simulink model "PFE_2Lignes_RNA (2)"  (R2024a)
settings: Solver=ode4  StartTime=0.0  StopTime=0.18  RelTol=1e-3
libraries: neural x202, spsRMSLib x12, spsThreePhasePISectionLineLib x4, spsThreePhaseFaultLib x2, spsThreePhaseVIMeasurementLib x2, spsThreePhaseSourceLib x2, spspowerguiLib x1
(part 5 of 10)

== system PFE_2Lignes_RNA (2)/RNA_Classificateur/Layer 3/Delays 1 ==
  "p{3}" : Inport  PortDimensions=20
      mask Display: e = 0.06;c1 = [120 230 180]/255;c2 = ([120 230 180]+0)/(256+128);c3 = ([120 230 180]+128)/(256+128);patch([0 1 1 0],[0 0 1 1],c1);patch([0 1 1 1-e 1-e 0+e],[0 0 1 1-e 0+e 0+e],c2);patch([0 0 1 1-e 0+e 0+e],[0 1 1 1-e 1-e 0+e],c3);plot([0 1 1 0 0],[0 0 1 1 0]);
  mux : Mux  Inputs=1
      mask Display: e = 0.06;c1 = [120 150 230]/255;c2 = ([120 150 230]+0)/383;c3 = ([120 150 230]+128)/383;patch([0 1 1 0],[0 0 1 1],c1);patch([0 1 1 1-e 1-e 0+e],[0 0 1 1-e 0+e 0+e],c2);patch([0 0 1 1-e 0+e 0+e],[0 1 1 1-e 1-e 0+e],c3);plot([0 1 1 0 0],[0 0 1 1 0]);disp('Mux')
  "pd{3,2}" : Outport
      mask Display: e = 0.06;c1 = [120 230 180]/255;c2 = ([120 230 180]+0)/(256+128);c3 = ([120 230 180]+128)/(256+128);patch([0 1 1 0],[0 0 1 1],c1);patch([0 1 1 1-e 1-e 0+e],[0 0 1 1-e 0+e 0+e],c2);patch([0 0 1 1-e 0+e 0+e],[0 1 1 1-e 1-e 0+e],c3);plot([0 1 1 0 0],[0 0 1 1 0]);
  wires:
  "p{3}"/1 -> mux/1
  mux/1 -> "pd{3,2}"/1

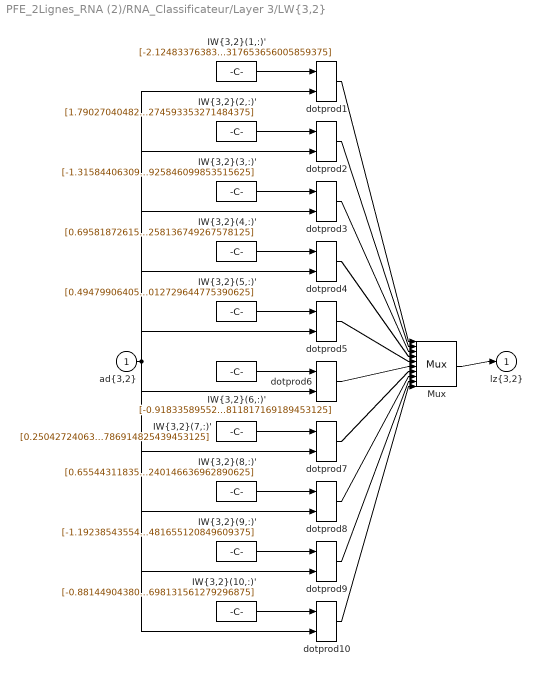
== system PFE_2Lignes_RNA (2)/RNA_Classificateur/Layer 3/LW{3,2} ==
  "ad{3,2}" : Inport  PortDimensions=20
      mask Display: e = 0.06;c1 = [120 230 180]/255;c2 = ([120 230 180]+0)/(256+128);c3 = ([120 230 180]+128)/(256+128);patch([0 1 1 0],[0 0 1 1],c1);patch([0 1 1 1-e 1-e 0+e],[0 0 1 1-e 0+e 0+e],c2);patch([0 0 1 1-e 0+e 0+e],[0 1 1 1-e 1-e 0+e],c3);plot([0 1 1 0 0],[0 0 1 1 0]);
  "IW{3,2}(1,:)'" : Constant  Value=[-2.124833763838835043458175277919508516788482666015625;2.235095062674105736988394710351713001728057861328125;-1.495799673223132675303759242524392902851104736328125;-0.10326184150683544171744898676479351706802845001220703125;0.30461440661710204036438653929508291184902191162109375;1.7655833119941684028475492596044205129146575927734375;-0.294301775431359435852840533698326908051967620849609375;1.422921443728915935622580946073867380619049072265625;-1.0126081617278674951165839956956915557384490966796875;2.06139005636338179527911051991395652294158935546875;-1.42107797840496008490163148962892591953277587890625;-0.4665987521331393939050258268252946436405181884765625;-0.78123086378600870016697399478289298713207244873046875;-0.9638905255282874673383730623754672706127166748046875;0.11887587911221302039432856645362335257232189178466796875;0.1219190321385441311274888676052796654403209686279296875;0.7209704057204142646497757596080191433429718017578125;0.807266197382073169563909686985425651073455810546875;-1.1797771643987851053481108465348370373249053955078125;-0.2368631238857614729198530767462216317653656005859375]
      mask Display: e = 0.06;c1 = [120 150 230]/255;c2 = ([120 150 230]+0)/383;c3 = ([120 150 230]+128)/383;patch([0 1 1 0],[0 0 1 1],c1);patch([0 1 1 1-e 1-e 0+e],[0 0 1 1-e 0+e 0+e],c2);patch([0 0 1 1-e 0+e 0+e],[0 1 1 1-e 1-e 0+e],c3);plot([0 1 1 0 0],[0 0 1 1 0]);disp('weights');
  "IW{3,2}(10,:)'" : Constant  Value=[-0.88144904380601041271603435234283097088336944580078125;1.2959793842845128697405243656248785555362701416015625;1.3513640222311844585334483781480230391025543212890625;-0.44568678579454512611590644155512563884258270263671875;-0.485414780167485904183166667280602268874645233154296875;-0.7871810260425171623666074083303101360797882080078125;2.007996352418774943515700215357355773448944091796875;-0.37565487427648835971893959140288643538951873779296875;-1.0046399001899637415391453032498247921466827392578125;-0.64463016403909667584315457133925519883632659912109375;1.4514250561273047690491466710227541625499725341796875;-1.64089130459730281330621437518857419490814208984375;0.85543383350244595053624152569682337343692779541015625;0.266300186174826258866943362590973265469074249267578125;1.525362775288933381290235047345049679279327392578125;-1.0373978509685557458652738205273635685443878173828125;-0.189926019352055830413661396960378624498844146728515625;-0.51200224756051238017562354798428714275360107421875;0.72520479466617115971160956178209744393825531005859375;1.131488984637971650926147049176506698131561279296875]
      mask Display: e = 0.06;c1 = [120 150 230]/255;c2 = ([120 150 230]+0)/383;c3 = ([120 150 230]+128)/383;patch([0 1 1 0],[0 0 1 1],c1);patch([0 1 1 1-e 1-e 0+e],[0 0 1 1-e 0+e 0+e],c2);patch([0 0 1 1-e 0+e 0+e],[0 1 1 1-e 1-e 0+e],c3);plot([0 1 1 0 0],[0 0 1 1 0]);disp('weights');
  "IW{3,2}(2,:)'" : Constant  Value=[1.7902704048235531519850383119774051010608673095703125;-0.83301117298299443003628539372584782540798187255859375;-0.86812317640997616052800367469899356365203857421875;-0.61903270694970424781189421992166899144649505615234375;-1.0952786106124217102575357785099186003208160400390625;0.98637534583504626883865284980856813490390777587890625;2.1858479023867385393486983957700431346893310546875;0.967325919819800095211803636630065739154815673828125;0.75786317317939388971126390970312058925628662109375;-2.060200915980545222083719636430032551288604736328125;-1.4236157537296836306239811165141873061656951904296875;1.2433599401893744573754929660935886204242706298828125;0.05806739015085897459567121359214070253074169158935546875;0.0020380782368509021973412842498873942531645298004150390625;0.84058335857627441978223714613704942166805267333984375;1.35282448767321827887144536362029612064361572265625;0.2189926893955626285848126144628622569143772125244140625;-0.42231741579335657643667900629225187003612518310546875;1.436115452384581825384657349786721169948577880859375;-0.41474159462432014233712607165216468274593353271484375]
      mask Display: e = 0.06;c1 = [120 150 230]/255;c2 = ([120 150 230]+0)/383;c3 = ([120 150 230]+128)/383;patch([0 1 1 0],[0 0 1 1],c1);patch([0 1 1 1-e 1-e 0+e],[0 0 1 1-e 0+e 0+e],c2);patch([0 0 1 1-e 0+e 0+e],[0 1 1 1-e 1-e 0+e],c3);plot([0 1 1 0 0],[0 0 1 1 0]);disp('weights');
  "IW{3,2}(3,:)'" : Constant  Value=[-1.3158440630983820884836177356191910803318023681640625;-1.419656511869585191476517138653434813022613525390625;1.1800655789785725602314414572902023792266845703125;-0.719240970988912042827223558560945093631744384765625;-0.11943453151677159429500107989952084608376026153564453125;-1.9966258446750460020524542414932511746883392333984375;-2.37447351454145749727331349276937544345855712890625;-0.78258770171416525140983821984264068305492401123046875;1.0354694090954545959704091728781349956989288330078125;0.605154989361207373832485245657153427600860595703125;1.23491208175254296719458579900674521923065185546875;1.2582457853531112679235093310126103460788726806640625;-0.67352823452173193885528235114179551601409912109375;0.85550010884744087658049238598323427140712738037109375;-1.2449073010859830201724207654478959739208221435546875;-0.449245519413075999892726031248457729816436767578125;0.07641744133077221778904686289024539291858673095703125;-0.426118641723025659562296141302795149385929107666015625;1.7786706927411055634280501180910505354404449462890625;-0.68789532767131744694921735572279430925846099853515625]
      mask Display: e = 0.06;c1 = [120 150 230]/255;c2 = ([120 150 230]+0)/383;c3 = ([120 150 230]+128)/383;patch([0 1 1 0],[0 0 1 1],c1);patch([0 1 1 1-e 1-e 0+e],[0 0 1 1-e 0+e 0+e],c2);patch([0 0 1 1-e 0+e 0+e],[0 1 1 1-e 1-e 0+e],c3);plot([0 1 1 0 0],[0 0 1 1 0]);disp('weights');
  "IW{3,2}(4,:)'" : Constant  Value=[0.69581872615161532991123749525286257266998291015625;-2.475637159212695781462798549910075962543487548828125;-1.0133208738240877533343109462293796241283416748046875;0.433411808461749981091770678176544606685638427734375;1.437967549207739725858345991582609713077545166015625;2.081675820617252536948171837138943374156951904296875;0.52801372365134557895771649782545864582061767578125;1.610670852459428648018047169898636639118194580078125;0.424212418998134166425728608373901806771755218505859375;1.6976510238713957701151002765982411801815032958984375;-0.08330331033522976602601062268149689771234989166259765625;-0.2255126598263615667061543490490294061601161956787109375;-0.5215191203851128332047437652363441884517669677734375;0.8126804349301448571196715420228429138660430908203125;-1.1216344746556570211026837569079361855983734130859375;0.80258429428750144296600410598330199718475341796875;-0.149635019068319385926457698587910272181034088134765625;0.7331158653688760740152474681963212788105010986328125;-2.20447234463556807071427101618610322475433349609375;0.10647105238430194795729022416708176024258136749267578125]
      mask Display: e = 0.06;c1 = [120 150 230]/255;c2 = ([120 150 230]+0)/383;c3 = ([120 150 230]+128)/383;patch([0 1 1 0],[0 0 1 1],c1);patch([0 1 1 1-e 1-e 0+e],[0 0 1 1-e 0+e 0+e],c2);patch([0 0 1 1-e 0+e 0+e],[0 1 1 1-e 1-e 0+e],c3);plot([0 1 1 0 0],[0 0 1 1 0]);disp('weights');
  "IW{3,2}(5,:)'" : Constant  Value=[0.4947990640517490046335069564520381391048431396484375;-0.08974147974601327792942839778334018774330615997314453125;-2.51838547573669035983812136691994965076446533203125;0.78890353171497540341050580536830238997936248779296875;0.35061679481755636533790720932302065193653106689453125;-1.480376772388819262005199561826884746551513671875;0.652323017941430549626602442003786563873291015625;-0.72082713149256083529081706728902645409107208251953125;1.6991012649264423117756450665183365345001220703125;-1.9962139405190624241726027321419678628444671630859375;0.996803418780932926068771848804317414760589599609375;0.67143035398569905769505794523865915834903717041015625;0.55786683853744400973795336540206335484981536865234375;1.3026453567663189847536386878346092998981475830078125;-2.003703998866505298082074659760110080242156982421875;-0.2075362615699163082449985040511819534003734588623046875;0.326835903571095764963416741011315025389194488525390625;-0.70344268967010170623410658663487993180751800537109375;1.5489136525381568265657961092074401676654815673828125;-1.3458171453073044521175916088395752012729644775390625]
      mask Display: e = 0.06;c1 = [120 150 230]/255;c2 = ([120 150 230]+0)/383;c3 = ([120 150 230]+128)/383;patch([0 1 1 0],[0 0 1 1],c1);patch([0 1 1 1-e 1-e 0+e],[0 0 1 1-e 0+e 0+e],c2);patch([0 0 1 1-e 0+e 0+e],[0 1 1 1-e 1-e 0+e],c3);plot([0 1 1 0 0],[0 0 1 1 0]);disp('weights');
  "IW{3,2}(6,:)'" : Constant  Value=[-0.918335895522720324635201905039139091968536376953125;-0.06660288456244077559542660083025111816823482513427734375;0.521999995099642344342782962485216557979583740234375;0.312043139980553829726517278686515055596828460693359375;-0.6648828394938106622902296294341795146465301513671875;0.626055990822066643630705584655515849590301513671875;-2.417297603923924231850151045364327728748321533203125;-1.9233356378126267305361807302688248455524444580078125;-2.43201499947078136898426237166859209537506103515625;2.0584786190281700868354164413176476955413818359375;1.117431727075297143159104962251149117946624755859375;0.7891952698726216741675898447283543646335601806640625;0.49732545500034597285576865033362992107868194580078125;0.2094270094966076134479493475737399421632289886474609375;-2.42116929455176244090353065985254943370819091796875;0.0618431619365222562390016491917776875197887420654296875;0.7995461321789729680631353403441607952117919921875;-0.11918414873537795661828653237535036168992519378662109375;0.63089454283535750800382402303512208163738250732421875;-0.87381958530518222261207483825273811817169189453125]
      mask Display: e = 0.06;c1 = [120 150 230]/255;c2 = ([120 150 230]+0)/383;c3 = ([120 150 230]+128)/383;patch([0 1 1 0],[0 0 1 1],c1);patch([0 1 1 1-e 1-e 0+e],[0 0 1 1-e 0+e 0+e],c2);patch([0 0 1 1-e 0+e 0+e],[0 1 1 1-e 1-e 0+e],c3);plot([0 1 1 0 0],[0 0 1 1 0]);disp('weights');
  "IW{3,2}(7,:)'" : Constant  Value=[0.250427240632494108041328217950649559497833251953125;-2.08025671431218039941768438438884913921356201171875;2.42990707620046375581068787141703069210052490234375;0.11455994775301982235848896607421920634806156158447265625;0.6406475041835746342400170760811306536197662353515625;0.51763219960940887176548130810260772705078125;0.470536791977866741820690776876290328800678253173828125;-0.70272121179415025782333259485312737524509429931640625;-1.224608169923931288991525434539653360843658447265625;0.050393218274616617680106145371610182337462902069091796875;-1.58937986271820452799374834285117685794830322265625;-2.157964013356698185219784136279486119747161865234375;0.62070509611624158363696324158809147775173187255859375;-0.818077207754040358622660278342664241790771484375;-0.315442098304872242664487203001044690608978271484375;-1.1224416867800073305261321365833282470703125;-0.463141270830716766937484862864948809146881103515625;0.607118804847790016765429754741489887237548828125;-0.81931020192715220407109200095874257385730743408203125;-1.62489586260114737825688280281610786914825439453125]
      mask Display: e = 0.06;c1 = [120 150 230]/255;c2 = ([120 150 230]+0)/383;c3 = ([120 150 230]+128)/383;patch([0 1 1 0],[0 0 1 1],c1);patch([0 1 1 1-e 1-e 0+e],[0 0 1 1-e 0+e 0+e],c2);patch([0 0 1 1-e 0+e 0+e],[0 1 1 1-e 1-e 0+e],c3);plot([0 1 1 0 0],[0 0 1 1 0]);disp('weights');
  "IW{3,2}(8,:)'" : Constant  Value=[0.65544311835529267540323417051695287227630615234375;-0.2789558565747463081407886420493014156818389892578125;1.5122990690464679364168887332198210060596466064453125;0.9264243230732105427449596390943042933940887451171875;1.0348363914273785990616261187824420630931854248046875;-2.406897129772101351363744470290839672088623046875;2.552754422334099881908286988618783652782440185546875;1.7910638120862192312898741874960251152515411376953125;1.153169780236896979630500936764292418956756591796875;-1.742649933801931894095105235464870929718017578125;0.5591525528291894087118407696834765374660491943359375;1.4404332192647670840557339033694006502628326416015625;-1.0494334787303241096623196426662616431713104248046875;0.24401763728825909272046601472538895905017852783203125;0.7970887178833712116698961835936643183231353759765625;-1.5691518900776966205512508167885243892669677734375;-0.1374688821458338872094628868580912239849567413330078125;0.2368711171063467568753679870496853254735469818115234375;1.4691258577164152399063823395408689975738525390625;0.66901975928571355556329081082367338240146636962890625]
      mask Display: e = 0.06;c1 = [120 150 230]/255;c2 = ([120 150 230]+0)/383;c3 = ([120 150 230]+128)/383;patch([0 1 1 0],[0 0 1 1],c1);patch([0 1 1 1-e 1-e 0+e],[0 0 1 1-e 0+e 0+e],c2);patch([0 0 1 1-e 0+e 0+e],[0 1 1 1-e 1-e 0+e],c3);plot([0 1 1 0 0],[0 0 1 1 0]);disp('weights');
  "IW{3,2}(9,:)'" : Constant  Value=[-1.19238543554604259355755857541225850582122802734375;2.348682819434720681073258674587123095989227294921875;0.6632684315488155402107395275379531085491180419921875;-0.59958044006351218779826695026713423430919647216796875;-0.993767654646679599039771346724592149257659912109375;-0.65034506134804159760420816382975317537784576416015625;-3.00792228401965555661945472820661962032318115234375;-0.3888056272152191628066475459490902721881866455078125;-0.07332293524646950333423234269503154791891574859619140625;1.3337493610745989602861527600907720625400543212890625;1.7509694952227408126788077424862422049045562744140625;-0.1297888271771781842911508420002064667642116546630859375;0.311098666598722151110933964446303434669971466064453125;-0.1951654740410834476538326498484821058809757232666015625;2.509675770038253261873251176439225673675537109375;-0.286945423200950011644039250313653610646724700927734375;0.95327847225390793806099054563674144446849822998046875;-0.360694961729205620937221965505159460008144378662109375;-0.807464102302945629929809001623652875423431396484375;1.754570433629685677345833028084598481655120849609375]
      mask Display: e = 0.06;c1 = [120 150 230]/255;c2 = ([120 150 230]+0)/383;c3 = ([120 150 230]+128)/383;patch([0 1 1 0],[0 0 1 1],c1);patch([0 1 1 1-e 1-e 0+e],[0 0 1 1-e 0+e 0+e],c2);patch([0 0 1 1-e 0+e 0+e],[0 1 1 1-e 1-e 0+e],c3);plot([0 1 1 0 0],[0 0 1 1 0]);disp('weights');
  Mux : Mux  Inputs=10
      mask Display: e = 0.06;c1 = [120 150 230]/255;c2 = ([120 150 230]+0)/383;c3 = ([120 150 230]+128)/383;patch([0 1 1 0],[0 0 1 1],c1);patch([0 1 1 1-e 1-e 0+e],[0 0 1 1-e 0+e 0+e],c2);patch([0 0 1 1-e 0+e 0+e],[0 1 1 1-e 1-e 0+e],c3);plot([0 1 1 0 0],[0 0 1 1 0]);disp('Mux');
  dotprod{1..10} (10 alike) : neural/Weight Functions/dotprod
  "lz{3,2}" : Outport
      mask Display: e = 0.06;c1 = [120 230 180]/255;c2 = ([120 230 180]+0)/(256+128);c3 = ([120 230 180]+128)/(256+128);patch([0 1 1 0],[0 0 1 1],c1);patch([0 1 1 1-e 1-e 0+e],[0 0 1 1-e 0+e 0+e],c2);patch([0 0 1 1-e 0+e 0+e],[0 1 1 1-e 1-e 0+e],c3);plot([0 1 1 0 0],[0 0 1 1 0]);
  wires:
  "IW{3,2}(1,:)'"/1 -> dotprod1/1
  "ad{3,2}"/1 -> dotprod1/2, dotprod2/2, dotprod3/2, dotprod4/2, dotprod5/2, dotprod6/2, dotprod7/2, dotprod8/2, dotprod9/2, dotprod10/2
  dotprod1/1 -> Mux/1
  "IW{3,2}(2,:)'"/1 -> dotprod2/1
  dotprod2/1 -> Mux/2
  "IW{3,2}(3,:)'"/1 -> dotprod3/1
  dotprod3/1 -> Mux/3
  "IW{3,2}(4,:)'"/1 -> dotprod4/1
  dotprod4/1 -> Mux/4
  "IW{3,2}(5,:)'"/1 -> dotprod5/1
  dotprod5/1 -> Mux/5
  "IW{3,2}(6,:)'"/1 -> dotprod6/1
  dotprod6/1 -> Mux/6
  "IW{3,2}(7,:)'"/1 -> dotprod7/1
  dotprod7/1 -> Mux/7
  "IW{3,2}(8,:)'"/1 -> dotprod8/1
  dotprod8/1 -> Mux/8
  "IW{3,2}(9,:)'"/1 -> dotprod9/1
  dotprod9/1 -> Mux/9
  "IW{3,2}(10,:)'"/1 -> dotprod10/1
  dotprod10/1 -> Mux/10
  Mux/1 -> "lz{3,2}"/1

== system PFE_2Lignes_RNA (2)/RNA_Detecteur/Layer 1/Delays 1 ==
  "p{1}" : Inport  PortDimensions=12
      mask Display: e = 0.06;c1 = [120 230 180]/255;c2 = ([120 230 180]+0)/(256+128);c3 = ([120 230 180]+128)/(256+128);patch([0 1 1 0],[0 0 1 1],c1);patch([0 1 1 1-e 1-e 0+e],[0 0 1 1-e 0+e 0+e],c2);patch([0 0 1 1-e 0+e 0+e],[0 1 1 1-e 1-e 0+e],c3);plot([0 1 1 0 0],[0 0 1 1 0]);
  mux : Mux  Inputs=1
      mask Display: e = 0.06;c1 = [120 150 230]/255;c2 = ([120 150 230]+0)/383;c3 = ([120 150 230]+128)/383;patch([0 1 1 0],[0 0 1 1],c1);patch([0 1 1 1-e 1-e 0+e],[0 0 1 1-e 0+e 0+e],c2);patch([0 0 1 1-e 0+e 0+e],[0 1 1 1-e 1-e 0+e],c3);plot([0 1 1 0 0],[0 0 1 1 0]);disp('Mux')
  "pd{1,1}" : Outport
      mask Display: e = 0.06;c1 = [120 230 180]/255;c2 = ([120 230 180]+0)/(256+128);c3 = ([120 230 180]+128)/(256+128);patch([0 1 1 0],[0 0 1 1],c1);patch([0 1 1 1-e 1-e 0+e],[0 0 1 1-e 0+e 0+e],c2);patch([0 0 1 1-e 0+e 0+e],[0 1 1 1-e 1-e 0+e],c3);plot([0 1 1 0 0],[0 0 1 1 0]);
  wires:
  "p{1}"/1 -> mux/1
  mux/1 -> "pd{1,1}"/1

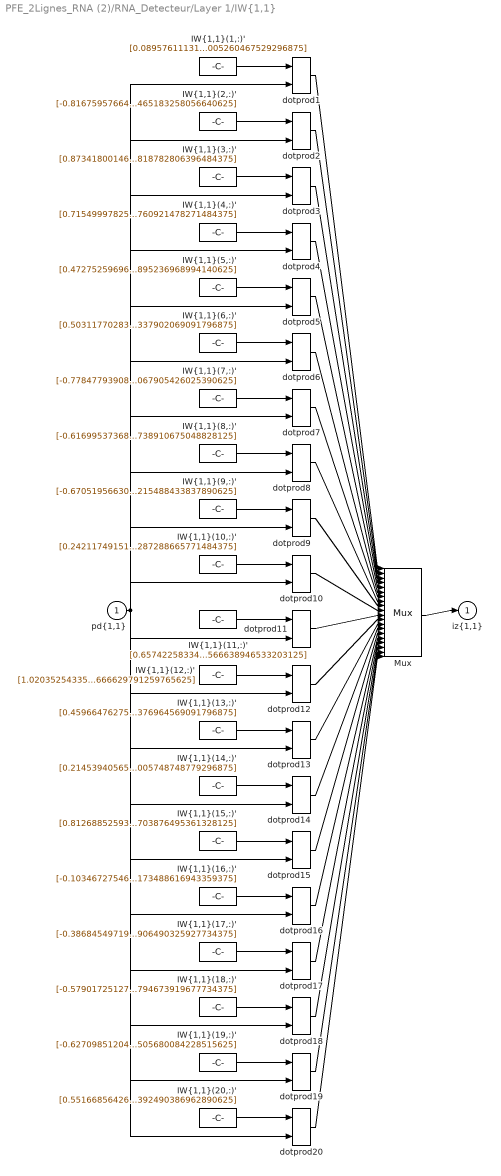
== system PFE_2Lignes_RNA (2)/RNA_Detecteur/Layer 1/IW{1,1} ==
  "pd{1,1}" : Inport  PortDimensions=12
      mask Display: e = 0.06;c1 = [120 230 180]/255;c2 = ([120 230 180]+0)/(256+128);c3 = ([120 230 180]+128)/(256+128);patch([0 1 1 0],[0 0 1 1],c1);patch([0 1 1 1-e 1-e 0+e],[0 0 1 1-e 0+e 0+e],c2);patch([0 0 1 1-e 0+e 0+e],[0 1 1 1-e 1-e 0+e],c3);plot([0 1 1 0 0],[0 0 1 1 0]);
  "IW{1,1}(1,:)'" : Constant  Value=[0.08957611131475044785599237684436957351863384246826171875;-0.65177834210718266216844085647608153522014617919921875;0.08211911108437659756464910287832026369869709014892578125;-0.346591794741859526851612827158533036708831787109375;0.88304376128066397466653825176763348281383514404296875;-0.026154692632130500939968698048687656410038471221923828125;0.586961087591081565051354118622839450836181640625;0.4489448684639676390162321695243008434772491455078125;-0.79399495629454375222877615669858641922473907470703125;-0.591077665620099335086479186429642140865325927734375;-0.251732194783920115721542742903693579137325286865234375;-0.65236339219162775560079126080381684005260467529296875]
      mask Display: e = 0.06;c1 = [120 150 230]/255;c2 = ([120 150 230]+0)/383;c3 = ([120 150 230]+128)/383;patch([0 1 1 0],[0 0 1 1],c1);patch([0 1 1 1-e 1-e 0+e],[0 0 1 1-e 0+e 0+e],c2);patch([0 0 1 1-e 0+e 0+e],[0 1 1 1-e 1-e 0+e],c3);plot([0 1 1 0 0],[0 0 1 1 0]);disp('Weights');
  "IW{1,1}(10,:)'" : Constant  Value=[0.2421174915169054531194348101053037680685520172119140625;-0.2574357370292668090172583106323145329952239990234375;0.7763225034072984698241270962171256542205810546875;-0.29577378432352829928930759706418029963970184326171875;-0.63148520046715861386843471336760558187961578369140625;0.0369141124621903127245303721792879514396190643310546875;0.68741061240758227768310462124645709991455078125;0.432043698966503075808986977790482342243194580078125;0.7895792067651121737270614175940863788127899169921875;0.42484176178848798155485155803035013377666473388671875;-0.72983865416340598653022198050166480243206024169921875;0.1178616038126195364466042292406200431287288665771484375]
      mask Display: e = 0.06;c1 = [120 150 230]/255;c2 = ([120 150 230]+0)/383;c3 = ([120 150 230]+128)/383;patch([0 1 1 0],[0 0 1 1],c1);patch([0 1 1 1-e 1-e 0+e],[0 0 1 1-e 0+e 0+e],c2);patch([0 0 1 1-e 0+e 0+e],[0 1 1 1-e 1-e 0+e],c3);plot([0 1 1 0 0],[0 0 1 1 0]);disp('Weights');
  "IW{1,1}(11,:)'" : Constant  Value=[0.65742258334486292081777492057881318032741546630859375;-0.1762033809634047376579957244757679291069507598876953125;-0.2358548113325060480160999532017740420997142791748046875;-0.63699842837748976709377757288166321814060211181640625;0.88508188672345589065315607513184659183025360107421875;0.593055855942936194225012513925321400165557861328125;0.53165849787483143717992106758174486458301544189453125;0.3422647416884441184947718284092843532562255859375;0.2304067220419007966381030882985214702785015106201171875;0.7758518669863441186151931105996482074260711669921875;0.48882514860545767110266979216248728334903717041015625;-0.1273918581133373362224148195309680886566638946533203125]
      mask Display: e = 0.06;c1 = [120 150 230]/255;c2 = ([120 150 230]+0)/383;c3 = ([120 150 230]+128)/383;patch([0 1 1 0],[0 0 1 1],c1);patch([0 1 1 1-e 1-e 0+e],[0 0 1 1-e 0+e 0+e],c2);patch([0 0 1 1-e 0+e 0+e],[0 1 1 1-e 1-e 0+e],c3);plot([0 1 1 0 0],[0 0 1 1 0]);disp('Weights');
  "IW{1,1}(12,:)'" : Constant  Value=[1.0203525433517339759958986178389750421047210693359375;0.03915050339096164122576482213844428770244121551513671875;-0.48216177591816766767607305155252106487751007080078125;-0.61393345445321434450391961945570074021816253662109375;0.531225038692037632159781423979438841342926025390625;-0.138360394973242428751092347738449461758136749267578125;0.32604544128300394500996617352939210832118988037109375;-0.553486149334765809015834747697226703166961669921875;-0.0122930968167403141533267074692048481665551662445068359375;-0.1606534945865641106355070633071591146290302276611328125;-0.7899348273056627789401318295858800411224365234375;0.52045213298950532276876401738263666629791259765625]
      mask Display: e = 0.06;c1 = [120 150 230]/255;c2 = ([120 150 230]+0)/383;c3 = ([120 150 230]+128)/383;patch([0 1 1 0],[0 0 1 1],c1);patch([0 1 1 1-e 1-e 0+e],[0 0 1 1-e 0+e 0+e],c2);patch([0 0 1 1-e 0+e 0+e],[0 1 1 1-e 1-e 0+e],c3);plot([0 1 1 0 0],[0 0 1 1 0]);disp('Weights');
  "IW{1,1}(13,:)'" : Constant  Value=[0.459664762757049205621484588846215046942234039306640625;0.7953238363826409251799987032427452504634857177734375;-0.1923194387721532672141933062448515556752681732177734375;0.2445980486996072456040707265856326557695865631103515625;0.4926456924184510199893338722176849842071533203125;-0.63444964774561818376952260223333723843097686767578125;0.396700572247033311779063069479889236390590667724609375;-0.424075135883652698520762669431860558688640594482421875;-0.60466124420165112685054964458686299622058868408203125;0.369478863100785093198652475621202029287815093994140625;0.6964931853581772802641580710769630968570709228515625;0.26938792359226215733514209205168299376964569091796875]
      mask Display: e = 0.06;c1 = [120 150 230]/255;c2 = ([120 150 230]+0)/383;c3 = ([120 150 230]+128)/383;patch([0 1 1 0],[0 0 1 1],c1);patch([0 1 1 1-e 1-e 0+e],[0 0 1 1-e 0+e 0+e],c2);patch([0 0 1 1-e 0+e 0+e],[0 1 1 1-e 1-e 0+e],c3);plot([0 1 1 0 0],[0 0 1 1 0]);disp('Weights');
  "IW{1,1}(14,:)'" : Constant  Value=[0.214539405656088033591544217415503226220607757568359375;-0.82824615002072976555069772075512446463108062744140625;0.7071282427336653686467116131098009645938873291015625;0.0681197815304366016686543616742710582911968231201171875;0.3203286122740951480380999782937578856945037841796875;-0.400985110996330773591722618220956064760684967041015625;-0.0203805885292373638317808826059263083152472972869873046875;-0.570802633192084130087096127681434154510498046875;0.77483392405658924051436997615383006632328033447265625;-0.5453417373401379109054687432944774627685546875;-0.346470469368322098180357215824187733232975006103515625;0.856406367680196733971342837321572005748748779296875]
      mask Display: e = 0.06;c1 = [120 150 230]/255;c2 = ([120 150 230]+0)/383;c3 = ([120 150 230]+128)/383;patch([0 1 1 0],[0 0 1 1],c1);patch([0 1 1 1-e 1-e 0+e],[0 0 1 1-e 0+e 0+e],c2);patch([0 0 1 1-e 0+e 0+e],[0 1 1 1-e 1-e 0+e],c3);plot([0 1 1 0 0],[0 0 1 1 0]);disp('Weights');
  "IW{1,1}(15,:)'" : Constant  Value=[0.81268852593549112395265865416149608790874481201171875;0.46638354297268802550746613633236847817897796630859375;0.9356160287932258068366309089469723403453826904296875;-0.04628300136490699767666257002929341979324817657470703125;0.25195908991665005860483006472350098192691802978515625;-0.1345428784789942378008475998285575769841670989990234375;-0.393349905794217968857395817394717596471309661865234375;-0.62418573246756048344963119234307669103145599365234375;-0.53978219315558251256703670151182450354099273681640625;0.58759853911462356368389237104565836489200592041015625;0.10499765777675425237891460028549772687256336212158203125;-0.475592235134400909135621304812957532703876495361328125]
      mask Display: e = 0.06;c1 = [120 150 230]/255;c2 = ([120 150 230]+0)/383;c3 = ([120 150 230]+128)/383;patch([0 1 1 0],[0 0 1 1],c1);patch([0 1 1 1-e 1-e 0+e],[0 0 1 1-e 0+e 0+e],c2);patch([0 0 1 1-e 0+e 0+e],[0 1 1 1-e 1-e 0+e],c3);plot([0 1 1 0 0],[0 0 1 1 0]);disp('Weights');
  "IW{1,1}(16,:)'" : Constant  Value=[-0.10346727546869809166718567894349689595401287078857421875;0.752439488931158084739081459701992571353912353515625;0.66711139814841480255580563607509247958660125732421875;-0.62668224757541401981342232829774729907512664794921875;-0.1058292027000466151154256522204377688467502593994140625;0.2437962030579083616554925129094044677913188934326171875;0.173481858436034475090536943753249943256378173828125;-0.1390647343226783239078514498032745905220508575439453125;-0.446067420652739243802642477021436206996440887451171875;-0.59891883895308717367100825867964886128902435302734375;-0.87075328239929439266830968335852958261966705322265625;-0.936143480536455907525805741897784173488616943359375]
      mask Display: e = 0.06;c1 = [120 150 230]/255;c2 = ([120 150 230]+0)/383;c3 = ([120 150 230]+128)/383;patch([0 1 1 0],[0 0 1 1],c1);patch([0 1 1 1-e 1-e 0+e],[0 0 1 1-e 0+e 0+e],c2);patch([0 0 1 1-e 0+e 0+e],[0 1 1 1-e 1-e 0+e],c3);plot([0 1 1 0 0],[0 0 1 1 0]);disp('Weights');
  "IW{1,1}(17,:)'" : Constant  Value=[-0.386845497193546272729491874997620470821857452392578125;-0.73850750780005014473061919488827697932720184326171875;0.65467651325997533451328536102664656937122344970703125;0.11210684405247468842237168473729980178177356719970703125;-0.760528669335034823717478502658195793628692626953125;0.424731464322543994516223619939410127699375152587890625;0.273598858580234860493618498367141000926494598388671875;-0.7395396911941392037448395058163441717624664306640625;-0.11088318973407072787207283681709668599069118499755859375;-0.169276557067893962393867468563257716596126556396484375;0.448312244327758124828875452294596470892429351806640625;0.6824135165594265028943254947080276906490325927734375]
      mask Display: e = 0.06;c1 = [120 150 230]/255;c2 = ([120 150 230]+0)/383;c3 = ([120 150 230]+128)/383;patch([0 1 1 0],[0 0 1 1],c1);patch([0 1 1 1-e 1-e 0+e],[0 0 1 1-e 0+e 0+e],c2);patch([0 0 1 1-e 0+e 0+e],[0 1 1 1-e 1-e 0+e],c3);plot([0 1 1 0 0],[0 0 1 1 0]);disp('Weights');
  "IW{1,1}(18,:)'" : Constant  Value=[-0.579017251273957089807709053275175392627716064453125;0.035288898206800763113211161225990508683025836944580078125;-0.484607301876166018939073865112732164561748504638671875;0.87892375948449219524860609453753568232059478759765625;-0.258431471551724190049981189076788723468780517578125;-0.65334251756482120132574209492304362356662750244140625;-0.262525450424333006704813442411250434815883636474609375;-0.69163816876343042761021706610335968434810638427734375;-0.172885601359937746135386760215624235570430755615234375;-0.35250777011847700403990302220336161553859710693359375;-0.54497431238440174894321899046190083026885986328125;0.63666002542588040480353583916439674794673919677734375]
      mask Display: e = 0.06;c1 = [120 150 230]/255;c2 = ([120 150 230]+0)/383;c3 = ([120 150 230]+128)/383;patch([0 1 1 0],[0 0 1 1],c1);patch([0 1 1 1-e 1-e 0+e],[0 0 1 1-e 0+e 0+e],c2);patch([0 0 1 1-e 0+e 0+e],[0 1 1 1-e 1-e 0+e],c3);plot([0 1 1 0 0],[0 0 1 1 0]);disp('Weights');
  "IW{1,1}(19,:)'" : Constant  Value=[-0.62709851204495670184968503235722891986370086669921875;-0.273774268969020351249810119043104350566864013671875;-0.67139813155045013903787776143872179090976715087890625;0.52471134920012030278257952886633574962615966796875;-0.01359355771396752489421633214305984438396990299224853515625;-0.78455326066255992589759671318461187183856964111328125;0.58866174288731898389670504911919124424457550048828125;0.30172706181111486056778403508360497653484344482421875;-0.573543662451698299520330692757852375507354736328125;-0.69487224064427610681349278820562176406383514404296875;0.0288657118790924538398456888899090699851512908935546875;0.363138139826928052489307674477458931505680084228515625]
      mask Display: e = 0.06;c1 = [120 150 230]/255;c2 = ([120 150 230]+0)/383;c3 = ([120 150 230]+128)/383;patch([0 1 1 0],[0 0 1 1],c1);patch([0 1 1 1-e 1-e 0+e],[0 0 1 1-e 0+e 0+e],c2);patch([0 0 1 1-e 0+e 0+e],[0 1 1 1-e 1-e 0+e],c3);plot([0 1 1 0 0],[0 0 1 1 0]);disp('Weights');
  "IW{1,1}(2,:)'" : Constant  Value=[-0.8167595766437625304234870782238431274890899658203125;-0.368034401202751604298413212745799683034420013427734375;0.38509081884209861446066724965930916368961334228515625;-0.62773189531141182495588282108656130731105804443359375;0.67052381424143281396510474223759956657886505126953125;-0.0981570967166232877243459142846404574811458587646484375;-0.79940889466730002954619749289122410118579864501953125;-0.32223091043541962630314401394571177661418914794921875;-0.444857906286153959030116311623714864253997802734375;0.1684032998891511478944948976277373731136322021484375;-0.050905698140885489999529767146668746136128902435302734375;0.007243607469497010710457463034117608913220465183258056640625]
      mask Display: e = 0.06;c1 = [120 150 230]/255;c2 = ([120 150 230]+0)/383;c3 = ([120 150 230]+128)/383;patch([0 1 1 0],[0 0 1 1],c1);patch([0 1 1 1-e 1-e 0+e],[0 0 1 1-e 0+e 0+e],c2);patch([0 0 1 1-e 0+e 0+e],[0 1 1 1-e 1-e 0+e],c3);plot([0 1 1 0 0],[0 0 1 1 0]);disp('Weights');
  "IW{1,1}(20,:)'" : Constant  Value=[0.55166856426260524326465883859782479703426361083984375;0.63442068387117200867209021453163586556911468505859375;-0.64551975846777354117733693783520720899105072021484375;0.33268348800567715262133106080000288784503936767578125;0.5696996516417425215905723234754987061023712158203125;0.1981947812236441730515679182644817046821117401123046875;-0.67340605986072443744916427021962590515613555908203125;0.51596893113867992042287369258701801300048828125;0.350311681159599264123727380138006992638111114501953125;0.86969636216077805812574297306127846240997314453125;0.5140031975612895376315236717346124351024627685546875;0.09087545484092053593716542536640190519392490386962890625]
      mask Display: e = 0.06;c1 = [120 150 230]/255;c2 = ([120 150 230]+0)/383;c3 = ([120 150 230]+128)/383;patch([0 1 1 0],[0 0 1 1],c1);patch([0 1 1 1-e 1-e 0+e],[0 0 1 1-e 0+e 0+e],c2);patch([0 0 1 1-e 0+e 0+e],[0 1 1 1-e 1-e 0+e],c3);plot([0 1 1 0 0],[0 0 1 1 0]);disp('Weights');
  "IW{1,1}(3,:)'" : Constant  Value=[0.87341800146215409217376191008952446281909942626953125;0.63240349531068373867270793198258616030216217041015625;-0.0901298486437955848060710195568390190601348876953125;0.1706747346413889088179161035441211424767971038818359375;0.20065395999648483194022219322505407035350799560546875;-0.7722637911239293995180332785821519792079925537109375;0.311576250000229648673411020354251377284526824951171875;0.54110975202710687170792880351655185222625732421875;-0.5844513542835787500706601349520497024059295654296875;0.55727872036100534192115674159140326082706451416015625;0.044462212427220114407955264823613106273114681243896484375;-0.53826036527788845287290087071596644818782806396484375]
      mask Display: e = 0.06;c1 = [120 150 230]/255;c2 = ([120 150 230]+0)/383;c3 = ([120 150 230]+128)/383;patch([0 1 1 0],[0 0 1 1],c1);patch([0 1 1 1-e 1-e 0+e],[0 0 1 1-e 0+e 0+e],c2);patch([0 0 1 1-e 0+e 0+e],[0 1 1 1-e 1-e 0+e],c3);plot([0 1 1 0 0],[0 0 1 1 0]);disp('Weights');
  "IW{1,1}(4,:)'" : Constant  Value=[0.7154999782523028262204434213344939053058624267578125;-0.28273330438534127750926927546970546245574951171875;0.239403400103008479060662239135126583278179168701171875;-0.186943212005827863464446636498905718326568603515625;-0.81655162913177792294305845643975771963596343994140625;-0.84598545272541014750089516383013688027858734130859375;0.3542638860406615020082199407625012099742889404296875;-0.08913753520304916466709954647740232758224010467529296875;0.71702942060983854144495808213832788169384002685546875;-0.51677745162800814426873330376110970973968505859375;-0.63550244591217486256340407635434530675411224365234375;0.40179575375678966420167625983594916760921478271484375]
      mask Display: e = 0.06;c1 = [120 150 230]/255;c2 = ([120 150 230]+0)/383;c3 = ([120 150 230]+128)/383;patch([0 1 1 0],[0 0 1 1],c1);patch([0 1 1 1-e 1-e 0+e],[0 0 1 1-e 0+e 0+e],c2);patch([0 0 1 1-e 0+e 0+e],[0 1 1 1-e 1-e 0+e],c3);plot([0 1 1 0 0],[0 0 1 1 0]);disp('Weights');
  "IW{1,1}(5,:)'" : Constant  Value=[0.47275259696093741013100952841341495513916015625;0.95191980835059275545262380546773783862590789794921875;-0.267477272524625442340351355596794746816158294677734375;0.431349317446108770912616137138684280216693878173828125;-0.83541659626972941676825712420395575463771820068359375;0.284360502383325997044494215515442192554473876953125;-0.155249089486058144959912397098378278315067291259765625;0.6354575555804882203148054031771607697010040283203125;0.495458990707767721328735888164374046027660369873046875;0.23832783664873991025245913988328538835048675537109375;-0.45940566270124649772554903393029235303401947021484375;0.4310465159422920411458335365750826895236968994140625]
      mask Display: e = 0.06;c1 = [120 150 230]/255;c2 = ([120 150 230]+0)/383;c3 = ([120 150 230]+128)/383;patch([0 1 1 0],[0 0 1 1],c1);patch([0 1 1 1-e 1-e 0+e],[0 0 1 1-e 0+e 0+e],c2);patch([0 0 1 1-e 0+e 0+e],[0 1 1 1-e 1-e 0+e],c3);plot([0 1 1 0 0],[0 0 1 1 0]);disp('Weights');
  "IW{1,1}(6,:)'" : Constant  Value=[0.5031177028379187898821101043722592294216156005859375;-0.42802091698753097492868846529745496809482574462890625;-0.77093577274295277401705561715061776340007781982421875;-0.53477250879138427119841026069479994475841522216796875;-0.61909541847356075461306090801372192800045013427734375;-0.36257203568845353114369345348677597939968109130859375;0.50236119648295785022895643123774789273738861083984375;-0.2926564045797250823710555778234265744686126708984375;0.0773278808985231880246402624834445305168628692626953125;0.5434026581720441395617626767489127814769744873046875;-0.4742551531192777947154581852373667061328887939453125;-0.37991087271973345007580746823805384337902069091796875]
      mask Display: e = 0.06;c1 = [120 150 230]/255;c2 = ([120 150 230]+0)/383;c3 = ([120 150 230]+128)/383;patch([0 1 1 0],[0 0 1 1],c1);patch([0 1 1 1-e 1-e 0+e],[0 0 1 1-e 0+e 0+e],c2);patch([0 0 1 1-e 0+e 0+e],[0 1 1 1-e 1-e 0+e],c3);plot([0 1 1 0 0],[0 0 1 1 0]);disp('Weights');
  "IW{1,1}(7,:)'" : Constant  Value=[-0.77847793908027063114474231042549945414066314697265625;0.08022723500615980274375260705710388720035552978515625;0.174012336459133554189548931390163488686084747314453125;0.448920870595960419535686014569364488124847412109375;-0.09027151553027255859174005081513314507901668548583984375;1.051382108758601052755921045900322496891021728515625;0.29165756079987958937493885969161055982112884521484375;-0.60621765387429527027762787838582880795001983642578125;-0.4100490606810840432672193855978548526763916015625;0.31677361452655594664662430659518577158451080322265625;0.0087531524014790966503607450022172997705638408660888671875;0.76868007080797406960215312210493721067905426025390625]
      mask Display: e = 0.06;c1 = [120 150 230]/255;c2 = ([120 150 230]+0)/383;c3 = ([120 150 230]+128)/383;patch([0 1 1 0],[0 0 1 1],c1);patch([0 1 1 1-e 1-e 0+e],[0 0 1 1-e 0+e 0+e],c2);patch([0 0 1 1-e 0+e 0+e],[0 1 1 1-e 1-e 0+e],c3);plot([0 1 1 0 0],[0 0 1 1 0]);disp('Weights');
  "IW{1,1}(8,:)'" : Constant  Value=[-0.616995373687099668558175835642032325267791748046875;-0.34791493540923046356994063899037428200244903564453125;-0.353155570556407616411576100290403701364994049072265625;-0.434762539767238498367163401780999265611171722412109375;-0.1883075975272310575991951964169857092201709747314453125;-0.46044396871365667056608117491123266518115997314453125;-0.8814615657090236755522028033738024532794952392578125;0.437413524205422510338081565350876189768314361572265625;0.55460228067132411045037088115350343286991119384765625;0.1927154021141372630676613653122331015765666961669921875;-0.385229319434725658855001029223785735666751861572265625;-0.80653235444588589064807138129253871738910675048828125]
      mask Display: e = 0.06;c1 = [120 150 230]/255;c2 = ([120 150 230]+0)/383;c3 = ([120 150 230]+128)/383;patch([0 1 1 0],[0 0 1 1],c1);patch([0 1 1 1-e 1-e 0+e],[0 0 1 1-e 0+e 0+e],c2);patch([0 0 1 1-e 0+e 0+e],[0 1 1 1-e 1-e 0+e],c3);plot([0 1 1 0 0],[0 0 1 1 0]);disp('Weights');
  "IW{1,1}(9,:)'" : Constant  Value=[-0.67051956630567577377632915158756077289581298828125;0.81600735468546592432659281257656402885913848876953125;0.00401482791638206083784101707578884088434278964996337890625;0.1810849328496317578451879626300069503486156463623046875;1.00294116975473546204966623918153345584869384765625;-0.308747165941168077996081819946994073688983917236328125;-0.05758841269461735523638168388060876168310642242431640625;-0.427485874122379982953390253896941430866718292236328125;-0.165248613357539986257194186691776849329471588134765625;-0.392865797977999087198242023077909834682941436767578125;-0.2486756511424098314844144397284253500401973724365234375;0.784123570559339899688211517059244215488433837890625]
      mask Display: e = 0.06;c1 = [120 150 230]/255;c2 = ([120 150 230]+0)/383;c3 = ([120 150 230]+128)/383;patch([0 1 1 0],[0 0 1 1],c1);patch([0 1 1 1-e 1-e 0+e],[0 0 1 1-e 0+e 0+e],c2);patch([0 0 1 1-e 0+e 0+e],[0 1 1 1-e 1-e 0+e],c3);plot([0 1 1 0 0],[0 0 1 1 0]);disp('Weights');
  Mux : Mux  Inputs=20
      mask Display: e = 0.06;c1 = [120 150 230]/255;c2 = ([120 150 230]+0)/383;c3 = ([120 150 230]+128)/383;patch([0 1 1 0],[0 0 1 1],c1);patch([0 1 1 1-e 1-e 0+e],[0 0 1 1-e 0+e 0+e],c2);patch([0 0 1 1-e 0+e 0+e],[0 1 1 1-e 1-e 0+e],c3);plot([0 1 1 0 0],[0 0 1 1 0]);disp('Mux');
  dotprod{1..20} (20 alike) : neural/Weight Functions/dotprod
  "iz{1,1}" : Outport
      mask Display: e = 0.06;c1 = [120 230 180]/255;c2 = ([120 230 180]+0)/(256+128);c3 = ([120 230 180]+128)/(256+128);patch([0 1 1 0],[0 0 1 1],c1);patch([0 1 1 1-e 1-e 0+e],[0 0 1 1-e 0+e 0+e],c2);patch([0 0 1 1-e 0+e 0+e],[0 1 1 1-e 1-e 0+e],c3);plot([0 1 1 0 0],[0 0 1 1 0]);
  wires:
  "IW{1,1}(1,:)'"/1 -> dotprod1/1
  "pd{1,1}"/1 -> dotprod1/2, dotprod2/2, dotprod3/2, dotprod4/2, dotprod5/2, dotprod6/2, dotprod7/2, dotprod8/2, dotprod9/2, dotprod10/2, dotprod11/2, dotprod12/2, dotprod13/2, dotprod14/2, dotprod15/2, dotprod16/2, dotprod17/2, dotprod18/2, dotprod19/2, dotprod20/2
  dotprod1/1 -> Mux/1
  "IW{1,1}(2,:)'"/1 -> dotprod2/1
  dotprod2/1 -> Mux/2
  "IW{1,1}(3,:)'"/1 -> dotprod3/1
  dotprod3/1 -> Mux/3
  "IW{1,1}(4,:)'"/1 -> dotprod4/1
  dotprod4/1 -> Mux/4
  "IW{1,1}(5,:)'"/1 -> dotprod5/1
  dotprod5/1 -> Mux/5
  "IW{1,1}(6,:)'"/1 -> dotprod6/1
  dotprod6/1 -> Mux/6
  "IW{1,1}(7,:)'"/1 -> dotprod7/1
  dotprod7/1 -> Mux/7
  "IW{1,1}(8,:)'"/1 -> dotprod8/1
  dotprod8/1 -> Mux/8
  "IW{1,1}(9,:)'"/1 -> dotprod9/1
  dotprod9/1 -> Mux/9
  "IW{1,1}(10,:)'"/1 -> dotprod10/1
  dotprod10/1 -> Mux/10
  "IW{1,1}(11,:)'"/1 -> dotprod11/1
  dotprod11/1 -> Mux/11
  "IW{1,1}(12,:)'"/1 -> dotprod12/1
  dotprod12/1 -> Mux/12
  "IW{1,1}(13,:)'"/1 -> dotprod13/1
  dotprod13/1 -> Mux/13
  "IW{1,1}(14,:)'"/1 -> dotprod14/1
  dotprod14/1 -> Mux/14
  "IW{1,1}(15,:)'"/1 -> dotprod15/1
  dotprod15/1 -> Mux/15
  "IW{1,1}(16,:)'"/1 -> dotprod16/1
  dotprod16/1 -> Mux/16
  "IW{1,1}(17,:)'"/1 -> dotprod17/1
  dotprod17/1 -> Mux/17
  "IW{1,1}(18,:)'"/1 -> dotprod18/1
  dotprod18/1 -> Mux/18
  "IW{1,1}(19,:)'"/1 -> dotprod19/1
  dotprod19/1 -> Mux/19
  "IW{1,1}(20,:)'"/1 -> dotprod20/1
  dotprod20/1 -> Mux/20
  Mux/1 -> "iz{1,1}"/1

== system PFE_2Lignes_RNA (2)/RNA_Detecteur/Layer 2/Delays 1 ==
  "p{2}" : Inport  PortDimensions=20
      mask Display: e = 0.06;c1 = [120 230 180]/255;c2 = ([120 230 180]+0)/(256+128);c3 = ([120 230 180]+128)/(256+128);patch([0 1 1 0],[0 0 1 1],c1);patch([0 1 1 1-e 1-e 0+e],[0 0 1 1-e 0+e 0+e],c2);patch([0 0 1 1-e 0+e 0+e],[0 1 1 1-e 1-e 0+e],c3);plot([0 1 1 0 0],[0 0 1 1 0]);
  mux : Mux  Inputs=1
      mask Display: e = 0.06;c1 = [120 150 230]/255;c2 = ([120 150 230]+0)/383;c3 = ([120 150 230]+128)/383;patch([0 1 1 0],[0 0 1 1],c1);patch([0 1 1 1-e 1-e 0+e],[0 0 1 1-e 0+e 0+e],c2);patch([0 0 1 1-e 0+e 0+e],[0 1 1 1-e 1-e 0+e],c3);plot([0 1 1 0 0],[0 0 1 1 0]);disp('Mux')
  "pd{2,1}" : Outport
      mask Display: e = 0.06;c1 = [120 230 180]/255;c2 = ([120 230 180]+0)/(256+128);c3 = ([120 230 180]+128)/(256+128);patch([0 1 1 0],[0 0 1 1],c1);patch([0 1 1 1-e 1-e 0+e],[0 0 1 1-e 0+e 0+e],c2);patch([0 0 1 1-e 0+e 0+e],[0 1 1 1-e 1-e 0+e],c3);plot([0 1 1 0 0],[0 0 1 1 0]);
  wires:
  "p{2}"/1 -> mux/1
  mux/1 -> "pd{2,1}"/1
